simulink model "PID_controller"  (R2022b)
settings: Solver=VariableStepAuto  StartTime=0.0  StopTime=50  RelTol=1e-3
settings Model: Creator=Dell  LastModifiedBy=Dell

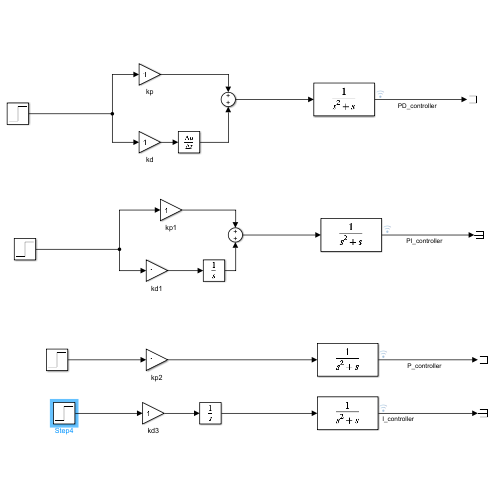
[thumbnail: Simulink's stored preview of the top-level diagram]
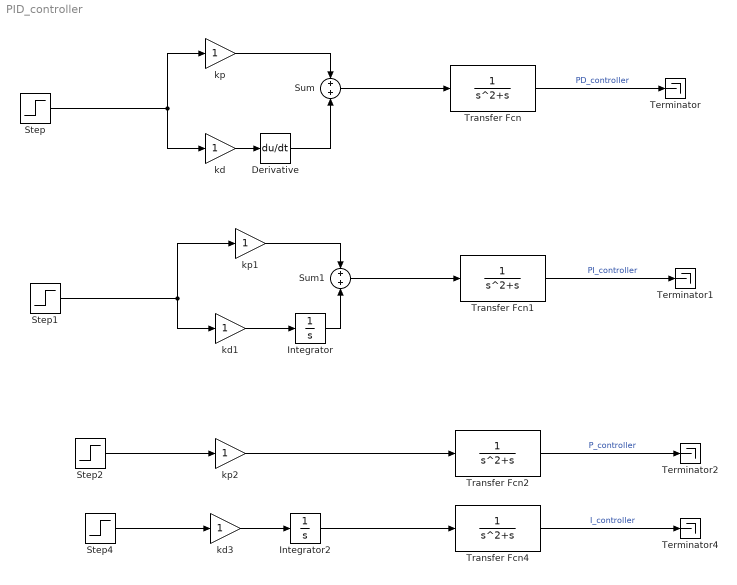
== system PID_controller ==
  Derivative : Derivative
  Integrator : Integrator
  Integrator2 : Integrator
  Step{,1..2,4} (4 alike) : Step  Time=10  SampleTime=0
  Sum : Sum
  Sum1 : Sum
  Terminator{,1..2,4} (4 alike) : Terminator
  Transfer Fcn{,1..2,4} (4 alike) : TransferFcn  Denominator=[1 1 0]
  kd : Gain
  kd1 : Gain
  kd3 : Gain
  kp : Gain
  kp1 : Gain
  kp2 : Gain
  wires:
  kd/1 -> Derivative/1
  kp/1 -> Sum/1
  Derivative/1 -> Sum/2
  Step/1 -> kd/1, kp/1
  kd1/1 -> Integrator/1
  Sum/1 -> Transfer Fcn/1
  Transfer Fcn/1 -> Terminator/1  "PD_controller"
  Transfer Fcn1/1 -> Terminator1/1  "PI_controller"
  Sum1/1 -> Transfer Fcn1/1
  Step1/1 -> kd1/1, kp1/1
  Integrator/1 -> Sum1/2
  kp1/1 -> Sum1/1
  Step2/1 -> kp2/1
  kp2/1 -> Transfer Fcn2/1
  Transfer Fcn2/1 -> Terminator2/1  "P_controller"
  Transfer Fcn4/1 -> Terminator4/1  "I_controller"
  kd3/1 -> Integrator2/1
  Step4/1 -> kd3/1
  Integrator2/1 -> Transfer Fcn4/1
